simulink model "MMC_1module_twist_20251006"  (R2024b)
settings: Solver=FixedStepAuto  StartTime=t_init_sim  StopTime=sim_time  FixedStep=Ts
model workspace (MAT data in the model file):
  Phs = Simulink.Parameter
  Phs.Complexity = 'real'
  Phs.Dimensions = [0 0]
  Phs.Description = 'Phase shift of the system'
  Phs.DataType = 'auto'
  Phs.DocUnits = 'degrees'
values from neighbouring files (symbols this model uses):
  C1low1_active = 1    [script_MMC_1module_twist_20251002.m]
  C2low1_active = 1    [script_MMC_1module_twist_20251002.m]
  expdelay = 0.00798    [script_MMC_1module_twist_20251002.m]
  f_HF_test = f_HF_tab(f_index)    [script_MMC_1module_twist_20251002.m]
  feeder_current_lower_rate_limit = -10    [script_MMC_1module_twist_20251002.m]    (also in twist_parameters.m = -500)
  feeder_current_upper_rate_limit = 0.386/(20e-3)    (= 19.3)    [twist_parameters.m]
  is6VExternallySupplied = false    [script_MMC_1module_twist_20251002.m]
  isFeederJumperOpen = false    [script_MMC_1module_twist_20251002.m]
  isHighFrequencyTest = false    [script_MMC_1module_twist_20251002.m]
  power_losses = false    [script_MMC_1module_twist_20251002.m]
  power_supply_C = 62.71e-2    (= 0.6271)    [script_MMC_1module_twist_20251002.m]
  power_supply_rC_down = 7.016e-2    (= 0.07016)    [script_MMC_1module_twist_20251002.m]
  power_supply_rC_up = 0.1    [script_MMC_1module_twist_20251002.m]
  R = 15    [MMC_parameters.m]
  Rdec = 15    [MMC_parameters.m]
  source_V = 0    [script_MMC_1module_twist_20251002.m]
  Ts = 1e-6    (= 1e-06)    [script_MMC_1module_twist_20251002.m]
  twist_data_acquisition_delay = 50e-9    (= 5e-08)    [script_MMC_1module_twist_20251002.m]
  twist_data_sampling_period = 1/twist_freq_data_sampling    (= 5e-05)    [script_MMC_1module_twist_20251002.m]
  twist_dead_time = 200e-9    (= 2e-07)    [twist_parameters.m]    (also in twist_parameters_before.m)
  twist_freq_switching = 200e3    (= 200000)    [twist_parameters.m]    (also in twist_parameters_before.m)
  twist_high_side_adc_R = 1/(1/2e6 + 1/2e6 + 1/(330e3+5.6e3))    (= 251272.836178)    [twist_parameters.m]    (also in twist_parameters_before.m = 335600)
  twist_high_side_C = 33e-6*4 + 4.7e-6*12    (= 0.0001884)    [twist_parameters.m]    (also in twist_parameters_before.m)
  twist_high_side_feeder_R = 47e3+4.7e3    (= 51700)    [twist_parameters.m]
  twist_high_side_rC = 0.1    [twist_parameters.m]    (also in twist_parameters_before.m)
  twist_low_side_adc_R = 150e3+470    (= 150470)    [twist_parameters.m]    (also in twist_parameters_before.m)
  twist_low_side_C_ceramic = 3*4.7e-6    (= 1.41e-05)    [twist_parameters.m]    (also in twist_parameters_before.m)
  twist_low_side_C_electrolytic = 47e-6    (= 4.7e-05)    [twist_parameters.m]    (also in twist_parameters_before.m)
  twist_low_side_L = 33e-6    (= 3.3e-05)    [twist_parameters.m]    (also in twist_parameters_before.m)
  twist_low_side_rC = 700e-3    (= 0.7)    [twist_parameters.m]    (also in twist_parameters_before.m = 0.35)
  twist_low_side_rL = 10e-3    (= 0.01)    [twist_parameters.m]    (also in twist_parameters_before.m)
  twist_R_VCC = (tau_VCC/twist_high_side_C  - twist_high_side_rC)/(1-(tau_VCC/twist_high_side_C - twist_high_side_rC)/R_parallel)    (= 1110.74997822)    [twist_parameters.m]
  VDC = 40    [MMC_parameters.m]
  Vdc_off_time = 0.4912    [script_MMC_1module_twist_20251002.m]
  Vdc_on_time = -0.0024    [script_MMC_1module_twist_20251002.m]
undefined symbols (not defined in the file or in its folder): C_SM, feeder_current, feeder_current_tab, gcbh, L_ac, power_supply_rC, sps_rtmsupport, twist_low_side_lC
libraries: spsSeriesRLCBranchLib x17, spsVoltageMeasurementLib x8, spsCurrentMeasurementLib x6, spsTriangleGeneratorLib x6, spsMosfetLib x6, spsIdealSwitchLib x4, spsDiodeLib x3, spsControlledCurrentSourceLib x3, spsGroundLib x1, spsControlledVoltageSourceLib x1, spspowerguiLib x1
(part 1 of 2)
settings Model: Creator=rodgeur  LastModifiedBy=ana
settings SolverCC: AlgebraicLoopSolver=TrustRegion
settings DataIOCC: SaveOutput=off  DSMLogging=off
settings DebuggingCC: AlgebraicLoopMsg=none  UnconnectedInputMsg=warning  UnconnectedOutputMsg=warning  UnconnectedLineMsg=warning  ArithmeticOperatorsInVariantConditions=warning
settings ModelReferenceCC: EnableRefExpFcnMdlSchedulingChecks=on
settings SFSimCC: CustomCodeUndefinedFunction=UseInterfaceOnly
settings RTWCC: GPUComputeCapability=3.5  DLArmComputeVersion=19.05

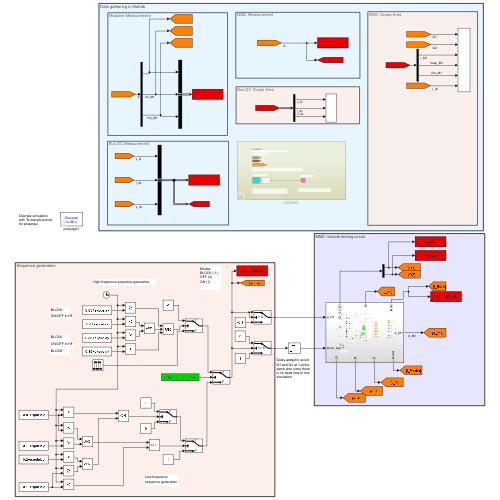
[thumbnail: Simulink's stored preview of the top-level diagram]
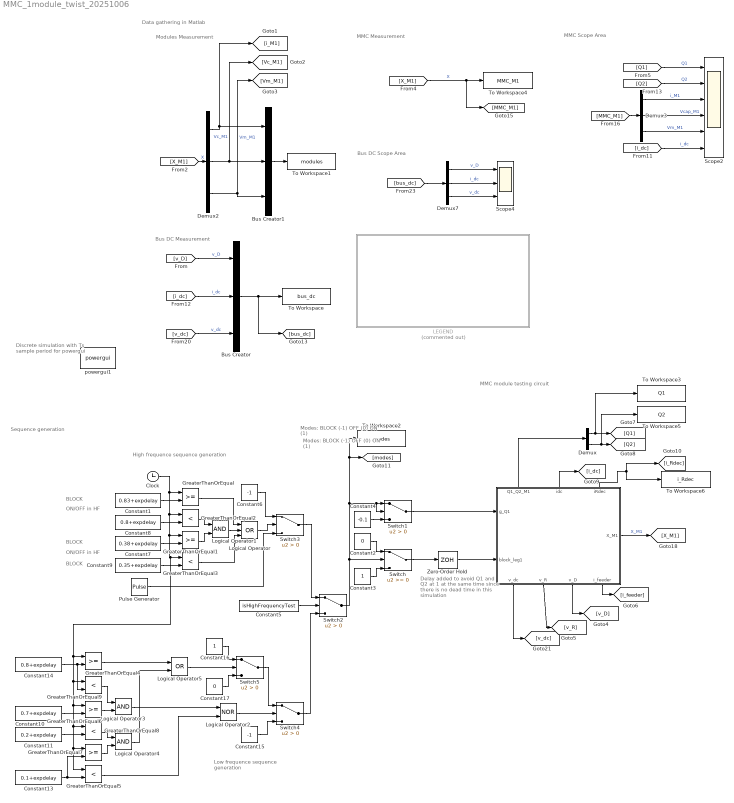
== system MMC_1module_twist_20251006 ==
  note: Modules Measurement
  note: Data gathering in Matlab
  note: MMC Measurement
  note: Bus DC Measurement
  note: MMC Scope Area
  note: MMC module testing circuit
  note: Bus DC Scope Area
  note: Sequence generation
  note: Delay added to avoid Q1 and Q2 at 1 at the same time since there is no dead time in this simulation
  note: Modes:
      | BLOCK (-1)
      | OFF (0)
      | ON (1)
  note: Modes:
      | BLOCK (-1)
      | OFF (0)
      | ON (1)
  note: High frequence sequence generation
  note: Discrete simulation with Ts sample period for powergui
  note: BLOCK
  note: BLOCK
  note: ON/OFF in HF
  note: BLOCK
  note: ON/OFF in HF
  note: Low frequence sequence generation
  " " : Subsystem
      settings: PortSchema="{\"entries\":[{\"content\":{\"sides\":[{\"content\":{\"connectorIds\":[\"In1\",\"In2\"]},\"type\":\"ConnectorPlacement.EquallySpacedRectSide\",\"uuid\":\"1684c177-0f69-459b-8ce9-190a6cc7c2f7\"},{\"content\":{\"connectorIds\":[\"Out1\"],\"side\":\"RIGHT\"},\"type\":\"ConnectorPlacement.EquallySpacedRectSide\",\"uuid\":\"0bff5431-30f2-45f3-9612-3e8ee114177b\"},{\"content\":{\"connectorIds\":[\"Out6\",\"Out7\",\"Out8\"],\"side\":\"TOP\"},\"type\":\"ConnectorPlacement.EquallySpacedRectSide\",\"uuid\":\"5880dbee-f5bf-4d11-b41f-6e883d19a036\"},{\"content\":{\"connectorIds\":[\"Out2\",\"Out3\",\"Out4\",\"Out5\"],\"side\":\"BOTTOM\"},\"type\":\"ConnectorPlacement.EquallySpacedRectSide\",\"uuid\":\"e7f28e42-6c15-4753-aad9-7fd8153dbb2b\"}]},\"type\":\"ConnectorPlacement.EquallySpacedConnector\",\"uuid\":\"d5dc9c97-4c49-4fa9-8e0e-631ade92c721\"}],\"packageUris\":[\"http://schema.mathworks.com/mf0/Connector/R2020b\"],\"version\":\"1.0\"}"
  Bus Creator : BusCreator  Inputs=3
  Bus Creator1 : BusCreator  Inputs=3
  Clock : Clock
  Constant1 : Constant  Value=0.83+expdelay
  Constant10 : Constant  Value=0.7+expdelay
  Constant11 : Constant  Value=0.2+expdelay
  Constant13 : Constant  Value=0.1+expdelay
  Constant14 : Constant  Value=0.8+expdelay
  Constant15 : Constant  Value=-1
  Constant16 : Constant
  Constant17 : Constant  Value=0
  Constant2 : Constant  Value=0
  Constant3 : Constant
  Constant4 : Constant  Value=-0.1
  Constant5 : Constant  Value=isHighFrequencyTest
  Constant6 : Constant  Value=-1
  Constant7 : Constant  Value=0.38+expdelay
  Constant8 : Constant  Value=0.8+expdelay
  Constant9 : Constant  Value=0.35+expdelay
  Demux : Demux  Outputs=2
  Demux2 : Demux  Outputs=3
  Demux3 : Demux  Outputs=3
  Demux7 : Demux  Outputs=3
  GreaterThanOrEqual{,1,4,6..7} (5 alike) : RelationalOperator  OutDataTypeStr=boolean  RndMeth=Simplest  InputSameDT=off
  GreaterThanOrEqual{2..3,5,8..9} (5 alike) : RelationalOperator  Operator=<  OutDataTypeStr=boolean  RndMeth=Simplest  InputSameDT=off
  LEGEND : Subsystem  Commented=on
  Logical Operator : Logic  Operator=OR  Inputs=3  AllPortsSameDT=off  OutDataTypeStr=boolean
  Logical Operator1 : Logic  AllPortsSameDT=off  OutDataTypeStr=boolean
  Logical Operator2 : Logic  Operator=NOR  AllPortsSameDT=off  OutDataTypeStr=boolean
  Logical Operator3 : Logic  AllPortsSameDT=off  OutDataTypeStr=boolean
  Logical Operator4 : Logic  AllPortsSameDT=off  OutDataTypeStr=boolean
  Logical Operator5 : Logic  Operator=OR  AllPortsSameDT=off  OutDataTypeStr=boolean
  Pulse Generator : DiscretePulseGenerator  Period=round(1/(f_HF_test*Ts))  PulseWidth=round(1/(f_HF_test*Ts*2))  PhaseDelay=round(((expdelay))/Ts)  SampleTime=Ts
  Scope2 : Scope  NumInputPorts=6
  Scope4 : Scope  NumInputPorts=3
  Switch : Switch  SaturateOnIntegerOverflow=off  InputSameDT=off
  Switch{1..5} (5 alike) : Switch  Criteria=u2 > Threshold  SaturateOnIntegerOverflow=off  InputSameDT=off
  To Workspace : ToWorkspace  VariableName=bus_dc  SaveFormat=Structure With Time  SampleTime=-1
  To Workspace1 : ToWorkspace  VariableName=modules  SaveFormat=Structure With Time  SampleTime=-1
  To Workspace2 : ToWorkspace  VariableName=modes  SaveFormat=Structure With Time  SampleTime=-1
  To Workspace3 : ToWorkspace  VariableName=Q1  SaveFormat=Structure With Time  SampleTime=-1
  To Workspace4 : ToWorkspace  VariableName=MMC_M1  SaveFormat=Structure With Time  SampleTime=-1
  To Workspace5 : ToWorkspace  VariableName=Q2  SaveFormat=Structure With Time  SampleTime=-1
  To Workspace6 : ToWorkspace  VariableName=i_Rdec  SaveFormat=Structure With Time  SampleTime=-1
  Zero-Order Hold : ZeroOrderHold  SampleTime=5*Ts
  powergui1 : spspowerguiLib/powergui  Priority=1  SimulationMode=Discrete  SampleTime=Ts  frequency=60  Iterations=50  frequencyindice=0  Pbase=100e6  ErrMax=1e-4  UnitsV=V  UnitsW=W  buscounter=0  FunctionMessages=off  echomessages=off  EnableUseOfTLC=off  CurrentSourceSwitches=off  DisableSnubberDevices=off  DisableRonSwitches=off  DisableVfSwitches=off  DisplayEquations=off  AutomaticDiscreteSolvers=off  SolverType=Backward Euler  Interpol=off  ExternalGateDelay=off  methode=off  Ts=0  x0status=blocks  SPID=off  SwTol=0  HookPort=off  NonlinearTolerance=1e-4  nMaxIteration=100  ContinueOnMaxIteration=off  RestoreLinks=warning  ResistiveCurrentMeasurement=off  Frange=[0:2:500]  Ylog=off  Xlog=on  ShowGrid=off  save=off  variable=ZData  structure=0  ZoomFFT=off  StartTime=0.0  cycles=1  DisplayStyle=1  fundamental=60  FreqAxis=off  MaxFrequency=1000  frequencyindicesteady=1  RmsSteady=1  display=off
  wires:
  Bus Creator1/1 -> To Workspace1/1
  Bus Creator/1 -> To Workspace/1, [bus_dc]
  [v_D] -> Bus Creator/1  "v_D"
  [v_dc] -> Bus Creator/3  "v_dc"
  [X_M1] -> [MMC_M1], To Workspace4/1  "X"
  " "/1(X_M1) -> [X_M1]  "X_M1"
  " "/2(v_dc) -> [v_dc]
  Demux3/2 -> Scope2/4  "Vcap_M1"
  Demux3/1 -> Scope2/3  "i_M1"
  Demux3/3 -> Scope2/5  "Vm_M1"
  [MMC_M1] -> Demux3/1
  [bus_dc] -> Demux7/1
  Demux7/1 -> Scope4/1  "v_D"
  Demux7/3 -> Scope4/3  "v_dc"
  [X_M1] -> Demux2/1  "X"
  Demux2/2 -> [Vc_M1], Bus Creator1/2  "Vc_M1"
  Demux2/3 -> [Vm_M1], Bus Creator1/3  "Vm_M1"
  Demux2/1 -> Bus Creator1/1, [i_M1]
  " "/3(v_R) -> [v_R]
  " "/4(v_D) -> [v_D]
  " "/5(i_feeder) -> [i_feeder]
  [i_dc] -> Scope2/6  "i_dc"
  [i_dc] -> Bus Creator/2  "i_dc"
  Demux7/2 -> Scope4/2  "i_dc"
  Constant4/1 -> Switch1/3
  Constant2/1 -> Switch/1
  Constant5/1 -> Switch2/2
  Constant3/1 -> Switch/3
  Switch2/1 -> To Workspace2/1, [modes], Switch1/2, Switch1/1, Switch/2
  Switch1/1 -> " "/1(g_Q1)
  " "/6(Q1_Q2_M1) -> Demux/1
  Demux/1 -> To Workspace3/1, [Q1]
  Demux/2 -> To Workspace5/1, [Q2]
  [Q1] -> Scope2/1  "Q1"
  [Q2] -> Scope2/2  "Q2"
  " "/7(idc) -> [i_dc]
  Pulse Generator/1 -> Switch3/3
  Constant1/1 -> GreaterThanOrEqual/2
  Constant6/1 -> Switch3/1
  Switch3/1 -> Switch2/1
  Switch4/1 -> Switch2/3
  Logical Operator/1 -> Switch3/2
  GreaterThanOrEqual/1 -> Logical Operator/1
  Logical Operator1/1 -> Logical Operator/2
  GreaterThanOrEqual1/1 -> Logical Operator1/2
  Constant7/1 -> GreaterThanOrEqual1/2
  GreaterThanOrEqual2/1 -> Logical Operator1/1
  Constant8/1 -> GreaterThanOrEqual2/2
  Switch/1 -> Zero-Order Hold/1
  Zero-Order Hold/1 -> " "/2(block_leg1)
  " "/8(iRdec) -> To Workspace6/1, [i_Rdec]
  Constant9/1 -> GreaterThanOrEqual3/2
  GreaterThanOrEqual3/1 -> Logical Operator/3
  Constant15/1 -> Switch4/3
  Switch5/1 -> Switch4/1
  Logical Operator2/1 -> Switch4/2
  Logical Operator3/1 -> Logical Operator2/1
  GreaterThanOrEqual9/1 -> Logical Operator3/1
  GreaterThanOrEqual8/1 -> Logical Operator4/1
  Constant13/1 -> GreaterThanOrEqual7/2, GreaterThanOrEqual5/2
  Constant10/1 -> GreaterThanOrEqual6/2
  Constant16/1 -> Switch5/1
  GreaterThanOrEqual7/1 -> Logical Operator4/2
  Constant11/1 -> GreaterThanOrEqual8/2
  GreaterThanOrEqual5/1 -> Logical Operator2/2
  Logical Operator4/1 -> Logical Operator5/2
  Constant14/1 -> GreaterThanOrEqual9/2, GreaterThanOrEqual4/2
  Clock/1 -> GreaterThanOrEqual2/1, GreaterThanOrEqual7/1, GreaterThanOrEqual5/1, GreaterThanOrEqual8/1, GreaterThanOrEqual6/1, GreaterThanOrEqual9/1, GreaterThanOrEqual4/1, GreaterThanOrEqual3/1, GreaterThanOrEqual1/1, GreaterThanOrEqual/1
  Constant17/1 -> Switch5/3
  GreaterThanOrEqual6/1 -> Logical Operator3/2
  Logical Operator5/1 -> Switch5/2
  GreaterThanOrEqual4/1 -> Logical Operator5/1

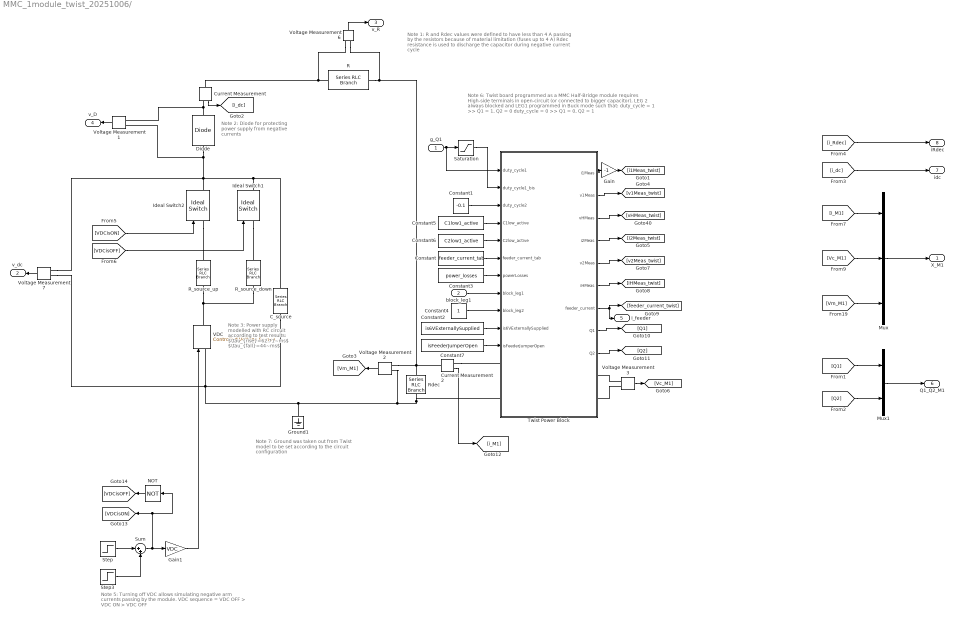
== system MMC_1module_twist_20251006/  ==
  note: Note 2:
      | Diode for protecting power supply from negative currents
  note: Note 3:
      | Power supply modelled with RC circuit according to test results:
      |
      | $\tau_{rise}=62.71~ms$
      | $\tau_{fall}=44~ms$
  note: Note 5:
      | Turning off VDC allows simulating negative arm currents passing by the module.
      |
      | VDC sequence = VDC OFF > VDC ON > VDC OFF
  note: Note 1:
      | R and Rdec values were defined to have less than 4 A passing by the resistors because of material limitation (fuses up to 4 A)
      |
      | Rdec resistance is used to discharge the capacitor during negative current cycle
  note: Note 6:
      | Twist board programmed as a MMC Half-Bridge module requires High-side terminals in open-circuit (or connected to bigger capacitor), LEG 2 always blocked and LEG1 programmed in Buck mode such that:
      |
      | duty_cycle = 1 >> Q1 = 1, Q2 = 0
      | duty_cycle = 0 >> Q1 = 0, Q2 = 1
  note: Note 7:
      | Ground was taken out from Twist model to be set according to the circuit configuration
  g_Q1 : Inport
  block_leg1 : Inport  Port=2
  C_source : spsSeriesRLCBranchLib/Series RLC Branch  LConnTagsString=__new0  RConnTagsString=__new0  BranchType=C  Resistance=power_supply_rC  Inductance=1e-3  SetiL0=off  InitialCurrent=0  Capacitance=power_supply_C  Setx0=on  InitialVoltage=0  Measurements=None
  Constant : Constant  Value=feeder_current_tab
  Constant1 : Constant  Value=-0.1
  Constant2 : Constant  Value=is6VExternallySupplied
  Constant3 : Constant  Value=power_losses
  Constant4 : Constant
  Constant5 : Constant  Value=C1low1_active
  Constant6 : Constant  Value=C2low1_active
  Constant7 : Constant  Value=isFeederJumperOpen
  Current Measurement : spsCurrentMeasurementLib/Current Measurement  PhasorSimulation=off  OutputType=Complex  PSBequivalent=0
  Current Measurement2 : spsCurrentMeasurementLib/Current Measurement  PhasorSimulation=off  OutputType=Complex  PSBequivalent=0
  Diode : spsDiodeLib/Diode  Ron=0.325  Lon=0  Vf=0.4404  IC=0  UseSnubber=0  Rs=500  Cs=250e-9  Measurements=off
  Gain : Gain  Gain=-1
  Gain1 : Gain  Gain=VDC
  Ground1 : spsGroundLib/Ground  LConnTagsString=a
  Ideal Switch1 : spsIdealSwitchLib/Ideal Switch  Ron=0.001  Lon=0  IC=0  Rs=1e5  Cs=inf  Measurements=on
  Ideal Switch2 : spsIdealSwitchLib/Ideal Switch  Ron=0.001  Lon=0  IC=0  Rs=1e5  Cs=inf  Measurements=on
  Mux : Mux  Inputs=3
  Mux1 : Mux  Inputs=2
  NOT : Logic  Operator=NOT  IconShape=distinctive  AllPortsSameDT=off  OutDataTypeStr=boolean
  R : spsSeriesRLCBranchLib/Series RLC Branch  LConnTagsString=__new0  RConnTagsString=__new0  BranchType=R  Resistance=R  Inductance=L_ac  SetiL0=off  InitialCurrent=0  Capacitance=C_SM  Setx0=off  InitialVoltage=0  Measurements=None
  R_source_down : spsSeriesRLCBranchLib/Series RLC Branch  LConnTagsString=__new0  RConnTagsString=__new0  BranchType=R  Resistance=power_supply_rC_down  Inductance=1e-3  SetiL0=off  InitialCurrent=0  Capacitance=power_supply_C  Setx0=off  InitialVoltage=0  Measurements=None
  R_source_up : spsSeriesRLCBranchLib/Series RLC Branch  LConnTagsString=__new0  RConnTagsString=__new0  BranchType=R  Resistance=power_supply_rC_up  Inductance=1e-3  SetiL0=off  InitialCurrent=0  Capacitance=power_supply_C  Setx0=off  InitialVoltage=0  Measurements=None
  Rdec : spsSeriesRLCBranchLib/Series RLC Branch  LConnTagsString=__new0  RConnTagsString=__new0  BranchType=R  Resistance=Rdec  Inductance=L_ac  SetiL0=off  InitialCurrent=0  Capacitance=C_SM  Setx0=off  InitialVoltage=0  Measurements=None
  Saturation : Saturate  UpperLimit=1  LowerLimit=0
  Step : Step  Time=Vdc_off_time  Before=1  After=0  SampleTime=0
  Step3 : Step  Time=Vdc_on_time  Before=-1  After=0  SampleTime=0
  Sum : Sum  Inputs=|++
  Twist Power Block : Subsystem
  VDC : spsControlledVoltageSourceLib/Controlled Voltage Source  Initialize=on  Source_Type=DC  Amplitude=VDC  Phase=0  Frequency=0  Measurements=None
  Voltage Measurement{1..3,6..7} (5 alike) : spsVoltageMeasurementLib/Voltage Measurement  PhasorSimulation=off  OutputType=Complex  PSBequivalent=0
  X_M1 : Outport
  v_dc : Outport  Port=2
  v_R : Outport  Port=3
  v_D : Outport  Port=4
  i_feeder : Outport  Port=5
  Q1_Q2_M1 : Outport  Port=6
  idc : Outport  Port=7
  iRdec : Outport  Port=8
  wires:
  Voltage Measurement6/1 -> v_R/1
  Voltage Measurement7/1 -> v_dc/1
  Twist Power Block/2(v1Meas) -> [v1Meas_twist]
  Constant/1 -> Twist Power Block/6(feeder_current_tab)
  Twist Power Block/7(feeder_current) -> [feeder_current_twist], i_feeder/1
  Constant3/1 -> Twist Power Block/7(powerLosses)
  Constant1/1 -> Twist Power Block/3(duty_cycle2)
  Twist Power Block/6(iHMeas) -> [iHMeas_twist]
  Twist Power Block/5(v2Meas) -> [v2Meas_twist]
  Twist Power Block/3(vHMeas) -> [vHMeas_twist]
  g_Q1/1 -> Twist Power Block/1(duty_cycle1), Saturation/1
  Saturation/1 -> Twist Power Block/2(duty_cycle1_bis)
  Twist Power Block/1(i1Meas) -> Gain/1
  Gain/1 -> [i1Meas_twist]
  Voltage Measurement1/1 -> v_D/1
  Current Measurement/1 -> [i_dc]
  Voltage Measurement2/1 -> [Vm_M1]
  Voltage Measurement3/1 -> [Vc_M1]
  [Vc_M1] -> Mux/2
  [i_M1] -> Mux/1
  [Vm_M1] -> Mux/3
  Mux/1 -> X_M1/1
  block_leg1/1 -> Twist Power Block/8(block_leg1)
  Twist Power Block/8(Q1) -> [Q1]
  Twist Power Block/9(Q2) -> [Q2]
  [Q1] -> Mux1/1
  [Q2] -> Mux1/2
  Mux1/1 -> Q1_Q2_M1/1
  Current Measurement2/1 -> [i_M1]
  [i_dc] -> idc/1
  Step/1 -> Sum/1
  Step3/1 -> Sum/2
  [i_Rdec] -> iRdec/1
  Constant2/1 -> Twist Power Block/10(is6VExternallySupplied)
  Constant4/1 -> Twist Power Block/9(block_leg2)
  Sum/1 -> NOT/1, [VDCisON], Gain1/1
  Gain1/1 -> VDC/1
  [VDCisON] -> Ideal Switch2/1
  [VDCisOFF] -> Ideal Switch1/1
  NOT/1 -> [VDCisOFF]
  Twist Power Block/4(i2Meas) -> [i2Meas_twist]
  Constant5/1 -> Twist Power Block/4(C1low_active)
  Constant6/1 -> Twist Power Block/5(C2low_active)
  Constant7/1 -> Twist Power Block/11(isFeederJumperOpen)
  connections:
  Twist Power Block/LConn3 -- Voltage Measurement2/LConn2 -- Ground1/LConn1 -- VDC/LConn1 -- Voltage Measurement7/LConn2 -- C_source/RConn1 -- Rdec/RConn1
  Voltage Measurement6/LConn1 -- Current Measurement/LConn1 -- R/LConn1
  Diode/RConn1 -- Voltage Measurement1/LConn2 -- Current Measurement/RConn1
  Voltage Measurement3/LConn1 -- Twist Power Block/RConn1
  Voltage Measurement3/LConn2 -- Twist Power Block/RConn2
  Current Measurement2/RConn1 -- Twist Power Block/LConn1
  R/RConn1 -- Voltage Measurement6/LConn2 -- Voltage Measurement2/LConn1 -- Current Measurement2/LConn1 -- Rdec/LConn1
  R_source_up/RConn1 -- R_source_down/RConn1 -- VDC/RConn1
  Diode/LConn1 -- Ideal Switch1/RConn1 -- C_source/LConn1 -- Voltage Measurement7/LConn1 -- Ideal Switch2/RConn1 -- Voltage Measurement1/LConn1
  Ideal Switch2/LConn1 -- R_source_up/LConn1
  Ideal Switch1/LConn1 -- R_source_down/LConn1

== system MMC_1module_twist_20251006/LEGEND ==
  note: Note:
      | Name the signals going into the scope to faciliate reading
  note: Color Code for scope
  note: Color code for subsystems
  note: Note:
      | Small subsystems usually contain a reduced set of functions
      | Model blocks regroup several small subsystems
  note: Note: Please avoid using global variables.  Rather, create the appropriate input/output
      | port in your subsystem
  note: This is a block for standardize the creation of models in simulink
  note: Color Code for variables
  note: LEGEND
  Model Blocks : Subsystem
  Scope : Scope
  Small subsystem : Subsystem
  wires:
  Model Blocks/1(Output_Example) -> Scope/1  "signal_name"

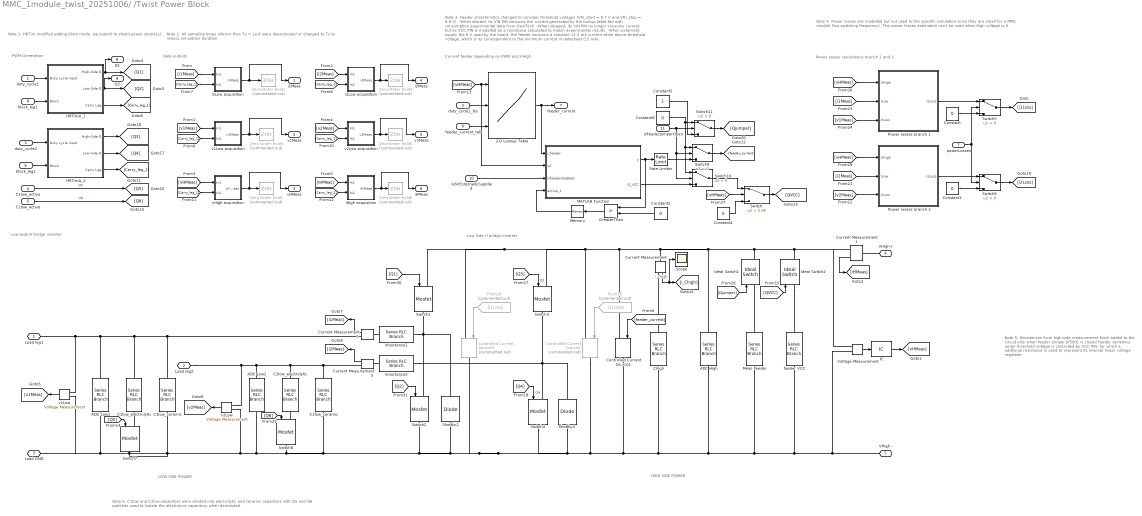
== system MMC_1module_twist_20251006/ /Twist Power Block ==
  note: Power losses calculations branch 1 and 2
  note: Current feeder depending on PWM and VHigh
  note: LOW SIDE POWER
  note: Data outputs
  note: PWM Generation
  note: Low-Side H bridge inverter
  note: Low Side H bridge inverter
  note: HIGH SIDE POWER
  note: Note 1:
      | HRTim modified adding block mode, equivalent to shield.power.stop(ALL);
  note: Note 2:
      | All sampling times inferior than Ts = 1e-6 were desactivated or changed to Ts to reduce simulation duration
  note: Note 3:
      | Feeder chracteristics changed to consider threshold voltages (Vth_start = 9.7 V and Vth_stop = 8.9 V).
      | -When started, its VIN PIN consums the current generated by the lookup table fed with consumption experimental data from OwnTech.
      | -When stopped, its VIN PIN no longer consums current but its VCC PIN is modelled as a resistance calculated to match experimental results.
      | -When externally supply the 6 V used by the board, the feeder consums a constant 11.2 mA current when above threshold voltage, which is its correspondent to the minimum current in datasheet (15 mA).
  note: Note 5:
      |
      | Resistances from high-side measurement block added to the circuit only when feeder jumper JP5001 is closed
      |
      | Feeder dynamics under threshold voltage is controlled by VCC PIN, for which a addtional resistance is used to represent its internal linear voltage regulator
  note: Note 4:
      | Power losses are modelled but not used in this specific simulation since they are small for a MMC module (low switching frequency).
      |
      | This power losses estimation can't be used when High voltage is 0.
  note: Note 6:
      | C1low and C2low capacitors were divided into electrolytic and ceramic capacitors with Q5 and Q6 switches used to isolate the electrolytic capacitors when demanded.
  duty_cycle1 : Inport
  duty_cycle1_bis : Inport  Port=2
  duty_cycle2 : Inport  Port=3
  C1low_active : Inport  Port=4
  C2low_active : Inport  Port=5
  feeder_current_tab : Inport  Port=6
  powerLosses : Inport  Port=7
  block_leg1 : Inport  Port=8
  block_leg2 : Inport  Port=9
  is6VExternallySupplied : Inport  Port=10
  isFeederJumperOpen : Inport  Port=11
  2-D Lookup Table : Lookup_n-D  LookupTableObject=feeder_current_tab  BreakpointsSpecification=Even spacing  BreakpointsForDimension1=[1:4]  BreakpointsForDimension2=[1:3]  BreakpointsForDimension1FirstPoint=feeder_VHigh_min  BreakpointsForDimension2FirstPoint=feeder_duty_min  BreakpointsForDimension1Spacing=feeder_VHigh_spacing  BreakpointsForDimension2Spacing=feeder_duty_spacing  TableSource=Input port  Table=feeder_current  InternalRulePriority=Speed  RndMeth=Simplest
      settings: InputPortMap=u0,u1,p221
  ADC High : spsSeriesRLCBranchLib/Series RLC Branch  LConnTagsString=__new0  RConnTagsString=__new0  BranchType=R  Resistance=twist_high_side_adc_R  Inductance=twist_low_side_L  SetiL0=off  InitialCurrent=0  Capacitance=1e-6  Setx0=off  InitialVoltage=0  Measurements=None
  ADC Low1 : spsSeriesRLCBranchLib/Series RLC Branch  LConnTagsString=__new0  RConnTagsString=__new0  BranchType=R  Resistance=twist_low_side_adc_R  Inductance=twist_low_side_L  SetiL0=off  InitialCurrent=0  Capacitance=1e-6  Setx0=off  InitialVoltage=0  Measurements=Branch voltage
  ADC Low2 : spsSeriesRLCBranchLib/Series RLC Branch  LConnTagsString=__new0  RConnTagsString=__new0  BranchType=R  Resistance=twist_low_side_adc_R  Inductance=twist_low_side_L  SetiL0=off  InitialCurrent=0  Capacitance=1e-6  Setx0=off  InitialVoltage=0  Measurements=Branch voltage
  C1low_ceramic : spsSeriesRLCBranchLib/Series RLC Branch  LConnTagsString=__new0  RConnTagsString=__new0  BranchType=C  Resistance=twist_low_side_rC  Inductance=1e-3  SetiL0=off  InitialCurrent=0  Capacitance=twist_low_side_C_ceramic  Setx0=off  InitialVoltage=0  Measurements=None
  C1low_electrolytic : spsSeriesRLCBranchLib/Series RLC Branch  LConnTagsString=__new0  RConnTagsString=__new0  BranchType=RC  Resistance=twist_low_side_rC  Inductance=twist_low_side_lC  SetiL0=off  InitialCurrent=0  Capacitance=twist_low_side_C_electrolytic  Setx0=off  InitialVoltage=0  Measurements=None
  C2low_ceramic : spsSeriesRLCBranchLib/Series RLC Branch  LConnTagsString=__new0  RConnTagsString=__new0  BranchType=C  Resistance=twist_low_side_rC  Inductance=1e-3  SetiL0=off  InitialCurrent=0  Capacitance=twist_low_side_C_ceramic  Setx0=off  InitialVoltage=0  Measurements=None
  C2low_electrolytic : spsSeriesRLCBranchLib/Series RLC Branch  LConnTagsString=__new0  RConnTagsString=__new0  BranchType=RC  Resistance=twist_low_side_rC  Inductance=twist_low_side_lC  SetiL0=off  InitialCurrent=0  Capacitance=twist_low_side_C_electrolytic  Setx0=off  InitialVoltage=0  Measurements=None
  Chigh : spsSeriesRLCBranchLib/Series RLC Branch  LConnTagsString=__new0  RConnTagsString=__new0  BranchType=RC  Resistance=twist_high_side_rC  Inductance=1e-3  SetiL0=off  InitialCurrent=0  Capacitance=twist_high_side_C  Setx0=on  InitialVoltage=source_V  Measurements=None
  Constant{,1..2,4,6} (5 alike) : Constant  Value=0
  Constant5 : Constant
  Controlled Current Source1 : spsControlledCurrentSourceLib/Controlled Current Source  Initialize=on  Source_Type=AC  Amplitude=0  Phase=0  Frequency=0  Measurements=None
  Controlled Current Source2 : spsControlledCurrentSourceLib/Controlled Current Source  Commented=on  Initialize=on  Source_Type=AC  Amplitude=0  Phase=0  Frequency=0  Measurements=None
  Controlled Current Source3 : spsControlledCurrentSourceLib/Controlled Current Source  Commented=on  Initialize=on  Source_Type=AC  Amplitude=0  Phase=0  Frequency=0  Measurements=None
  Current Measurement{,1,5..6} (4 alike) : spsCurrentMeasurementLib/Current Measurement  PhasorSimulation=off  OutputType=Complex  PSBequivalent=0
  From16 : From  Commented=on  GotoTag=i2Loss
  From28 : From  Commented=on  GotoTag=i1Loss
  GreaterThan : RelationalOperator  Operator=>  OutDataTypeStr=boolean  RndMeth=Simplest  InputSameDT=off
  HRTimA_1 : Subsystem
  HRTimA_2 : Subsystem
  IC : InitialCondition  Value=source_V
  Ideal Switch1 : spsIdealSwitchLib/Ideal Switch  Ron=0.001  Lon=0  IC=0  Rs=1e5  Cs=inf  Measurements=on
  Ideal Switch2 : spsIdealSwitchLib/Ideal Switch  Ron=0.001  Lon=0  IC=0  Rs=1e5  Cs=inf  Measurements=on
  Inductance1 : spsSeriesRLCBranchLib/Series RLC Branch  LConnTagsString=__new0  RConnTagsString=__new0  BranchType=RL  Resistance=twist_low_side_rL  Inductance=twist_low_side_L  SetiL0=off  InitialCurrent=0  Capacitance=1e-6  Setx0=off  InitialVoltage=0  Measurements=None
  Inductance2 : spsSeriesRLCBranchLib/Series RLC Branch  LConnTagsString=__new0  RConnTagsString=__new0  BranchType=RL  Resistance=twist_low_side_rL  Inductance=twist_low_side_L  SetiL0=off  InitialCurrent=0  Capacitance=1e-6  Setx0=off  InitialVoltage=0  Measurements=None
  MATLAB Function : MATLAB Function  TreatAsAtomicUnit=on
  Meas Feeder : spsSeriesRLCBranchLib/Series RLC Branch  LConnTagsString=__new0  RConnTagsString=__new0  BranchType=R  Resistance=twist_high_side_feeder_R  Inductance=twist_low_side_L  SetiL0=off  InitialCurrent=0  Capacitance=1e-6  Setx0=off  InitialVoltage=0  Measurements=None
  Memory : Memory  InheritSampleTime=on  LinearizeAsDelay=on
  Power losses branch 1 : Subsystem
  Power losses branch 2 : Subsystem
  Rate Limiter : RateLimiter  RisingSlewLimit=feeder_current_upper_rate_limit  FallingSlewLimit=feeder_current_lower_rate_limit  SampleTimeMode=inherited
  Scope : Scope
  Shottky2 : spsDiodeLib/Diode  Ron=twist_shottky_Ron  Lon=0  Vf=twist_shottky_Vf  IC=0  UseSnubber=0  Rs=twist_shottky_Rs  Cs=twist_shottky_Cs  Measurements=off
  Shottky4 : spsDiodeLib/Diode  Ron=twist_shottky_Ron  Lon=0  Vf=twist_shottky_Vf  IC=0  UseSnubber=0  Rs=twist_shottky_Rs  Cs=twist_shottky_Cs  Measurements=off
  Switch : Switch  Criteria=u2 > Threshold  Threshold=2.05  SaturateOnIntegerOverflow=off  InputSameDT=off
  Switch{1..4} (4 alike) : spsMosfetLib/Mosfet  Ron=twist_FET_Ron  Lon=0  Rd=twist_FET_Rd  Vfd=twist_FET_Vf  IC=0  Rs=twist_FET_Rs  Cs=twist_FET_Cs  Measurements=off
  Switch{5..6,9..11} (5 alike) : Switch  Criteria=u2 > Threshold  SaturateOnIntegerOverflow=off  InputSameDT=off
  Switch7 : spsMosfetLib/Mosfet  Ron=twist_FET_Clow_Ron  Lon=0  Rd=twist_FET_Clow_Ron  Vfd=0  IC=0  Rs=twist_FET_Rs  Cs=twist_FET_Cs  Measurements=off
  Switch8 : spsMosfetLib/Mosfet  Ron=twist_FET_Clow_Ron  Lon=0  Rd=twist_FET_Clow_Ron  Vfd=0  IC=0  Rs=twist_FET_Rs  Cs=twist_FET_Cs  Measurements=off
  Voltage Measurement : spsVoltageMeasurementLib/Voltage Measurement  PhasorSimulation=off  OutputType=Complex  PSBequivalent=0
  Zero-Order Hold{1..6} (6 alike) : ZeroOrderHold  Commented=on  SampleTime=twist_data_sampling_period
  feeder VCC : spsSeriesRLCBranchLib/Series RLC Branch  LConnTagsString=__new0  RConnTagsString=__new0  BranchType=R  Resistance=twist_R_VCC  Inductance=twist_low_side_L  SetiL0=off  InitialCurrent=0  Capacitance=1e-6  Setx0=off  InitialVoltage=0  Measurements=None
  i1Low acquisition : Subsystem
  i2Low acquisition : Subsystem
  iHigh acquisition : Subsystem
  v1Low : spsVoltageMeasurementLib/Voltage Measurement  PhasorSimulation=off  OutputType=Complex  PSBequivalent=0
  v1Low acquisition : Subsystem
  v2Low : spsVoltageMeasurementLib/Voltage Measurement  PhasorSimulation=off  OutputType=Complex  PSBequivalent=0
  v2Low acquisition : Subsystem
  vHigh acquisition : Subsystem
  Load leg1 : PMIOPort  Side=Left
  Load leg2 : PMIOPort  Port=2  Side=Left
  Load GND : PMIOPort  Port=3  Side=Left
  VHigh+ : PMIOPort  Port=4  Side=Right
  VHigh - : PMIOPort  Port=5  Side=Right
  i1Meas : Outport
  v1Meas : Outport  Port=2
  vHMeas : Outport  Port=3
  i2Meas : Outport  Port=4
  v2Meas : Outport  Port=5
  iHMeas : Outport  Port=6
  feeder_current : Outport  Port=7
  Q1 : Outport  Port=8
  Q2 : Outport  Port=9
  wires:
  duty_cycle1/1 -> HRTimA_1/1(Duty cycle input)
  HRTimA_1/2(Low-Side Q) -> [Q2], Q2/1
  [v1Meas] -> v1Low acquisition/1(In1)
  C1low_active/1 -> [Q5]  "Q5"
  HRTimA_1/1(High-Side Q) -> [Q1], Q1/1
  HRTimA_2/1(High-Side Q) -> [Q3]
  HRTimA_2/2(Low-Side Q) -> [Q4]
  [Carry_leg_1] -> vHigh acquisition/2(In2)
  [vHMeas] -> vHigh acquisition/1(In1)
  [i2Meas] -> i2Low acquisition/1(In1)
  [Carry_leg_2] -> i2Low acquisition/2(In2)
  [v2Meas] -> v2Low acquisition/1(In1)
  [Carry_leg_2] -> v2Low acquisition/2(In2)
  [iHMeas] -> iHigh acquisition/1(In1)
  [Carry_leg_2] -> iHigh acquisition/2(In2)
  [Carry_leg_1] -> v1Low acquisition/2(In2)
  v1Low acquisition/1(v1Meas) -> v1Meas/1, Zero-Order Hold3/1
  i2Low acquisition/1(i2Meas) -> i2Meas/1, Zero-Order Hold4/1
  v2Low acquisition/1(v2Meas) -> v2Meas/1, Zero-Order Hold5/1
  iHigh acquisition/1(iHMeas) -> iHMeas/1, Zero-Order Hold6/1
  vHigh acquisition/1(vHMeas) -> vHMeas/1, Zero-Order Hold2/1
  HRTimA_2/3(Carry Leg) -> [Carry_leg_2]
  HRTimA_1/3(Carry Leg) -> [Carry_leg_1]
  duty_cycle2/1 -> HRTimA_2/1(Duty cycle input)
  [vHMeas] -> MATLAB Function/2(vC), 2-D Lookup Table/1
  v2Low/1 -> [v2Meas]
  [Q3] -> Switch3/1  "Q3"
  Current Measurement6/1 -> [i1Meas]
  [Q1] -> Switch1/1
  [Q4] -> Switch4/1  "Q4"
  v1Low/1 -> [v1Meas]
  [Q2] -> Switch2/1
  Current Measurement1/1 -> [iHMeas]
  Current Measurement5/1 -> [i2Meas]
  [Carry_leg_1] -> i1Low acquisition/2(In2)
  [i1Meas] -> i1Low acquisition/1(In1)
  i1Low acquisition/1(i1Meas) -> i1Meas/1, Zero-Order Hold1/1
  Voltage Measurement/1 -> IC/1
  IC/1 -> [vHMeas]
  [vHMeas] -> Power losses branch 1/1(VHigh)
  [i1Meas] -> Power losses branch 1/2(ILow)
  [v1Meas] -> Power losses branch 1/3(VLow)
  Power losses branch 1/1(i1Loss) -> Switch5/1
  Switch5/1 -> [i1Loss]
  Constant/1 -> Switch5/3
  feeder_current_tab/1 -> 2-D Lookup Table/3
  duty_cycle1_bis/1 -> 2-D Lookup Table/2
  [Q5] -> Switch7/1
  C2low_active/1 -> [Q6]  "Q6"
  [feeder_current] -> Controlled Current Source1/1
  block_leg1/1 -> HRTimA_1/2(Block)
  Current Measurement/1 -> Scope/1, [i_Chigh]  "i_Chigh"
  block_leg2/1 -> HRTimA_2/2(Block)
  GreaterThan/1 -> Memory/1
  Constant2/1 -> GreaterThan/2
  [QVCC] -> Ideal Switch2/1
  2-D Lookup Table/1 -> feeder_current/1, MATLAB Function/1(i_feeder)
  MATLAB Function/1(y) -> GreaterThan/1, Rate Limiter/1
  powerLosses/1 -> Switch5/2, Switch6/2
  [vHMeas] -> Power losses branch 2/1(VHigh)
  [i2Meas] -> Power losses branch 2/2(ILow)
  [v2Meas] -> Power losses branch 2/3(VLow)
  Switch6/1 -> [i2Loss]
  Constant1/1 -> Switch6/3
  Power losses branch 2/1(i1Loss) -> Switch6/1
  is6VExternallySupplied/1 -> MATLAB Function/3(isfeederdisabled)
  Memory/1 -> MATLAB Function/4(active_1)
  [vHMeas] -> Switch/2
  Constant4/1 -> Switch/3
  [Q6] -> Switch8/1
  Switch9/1 -> [feeder_current]
  Rate Limiter/1 -> Switch9/3
  MATLAB Function/2(Q_VCC) -> Switch10/3
  Constant6/1 -> Switch11/1, Switch10/1, Switch9/1
  isFeederJumperOpen/1 -> Switch11/2, Switch9/2, Switch10/2
  Switch/1 -> [QVCC]
  Switch10/1 -> Switch/1
  Constant5/1 -> Switch11/3
  Switch11/1 -> [Qjumper]
  [Qjumper] -> Ideal Switch1/1
  From16/1 -> Controlled Current Source2/1
  From28/1 -> Controlled Current Source3/1
  connections:
  Inductance2/LConn1 -- Current Measurement5/LConn1
  Current Measurement6/LConn1 -- Inductance1/LConn1
  VHigh+/RConn1 -- Current Measurement1/LConn1
  v2Low/LConn1 -- Load leg2/RConn1 -- ADC Low2/LConn1 -- C2low_electrolytic/LConn1 -- C2low_ceramic/LConn1 -- Current Measurement5/RConn1
  Switch4/LConn1 -- Switch3/RConn1 -- Shottky4/RConn1 -- Inductance2/RConn1
  v1Low/LConn1 -- Load leg1/RConn1 -- C1low_ceramic/LConn1 -- Current Measurement6/RConn1 -- C1low_electrolytic/LConn1 -- ADC Low1/LConn1
  Current Measurement/RConn1 -- Chigh/LConn1
  ADC High/RConn1 -- Meas Feeder/RConn1 -- feeder VCC/RConn1 -- Voltage Measurement/LConn2 -- VHigh -/RConn1 -- Chigh/RConn1 -- Controlled Current Source2/RConn1 -- Controlled Current Source3/RConn1 -- Switch2/RConn1 -- Load GND/RConn1 -- v1Low/LConn2 -- ADC Low1/RConn1 -- Switch7/RConn1 -- C1low_ceramic/RConn1 -- v2Low/LConn2 -- ADC Low2/RConn1 -- Switch8/RConn1 -- C2low_ceramic/RConn1 -- Shottky2/LConn1 -- Switch4/RConn1 -- Shottky4/LConn1 -- Controlled Current Source1/RConn1
  Switch7/LConn1 -- C1low_electrolytic/RConn1
  Switch8/LConn1 -- C2low_electrolytic/RConn1
  Inductance1/RConn1 -- Shottky2/RConn1 -- Switch2/LConn1 -- Switch1/RConn1
  Ideal Switch2/LConn1 -- feeder VCC/LConn1
  Current Measurement/LConn1 -- Ideal Switch1/RConn1 -- Voltage Measurement/LConn1 -- Current Measurement1/RConn1 -- Ideal Switch2/RConn1 -- ADC High/LConn1 -- Controlled Current Source2/LConn1 -- Controlled Current Source3/LConn1 -- Switch1/LConn1 -- Switch3/LConn1 -- Controlled Current Source1/LConn1
  Meas Feeder/LConn1 -- Ideal Switch1/LConn1

== system MMC_1module_twist_20251006/LEGEND/Model Blocks ==
  Output_Example : Outport

== system MMC_1module_twist_20251006/LEGEND/Small subsystem ==

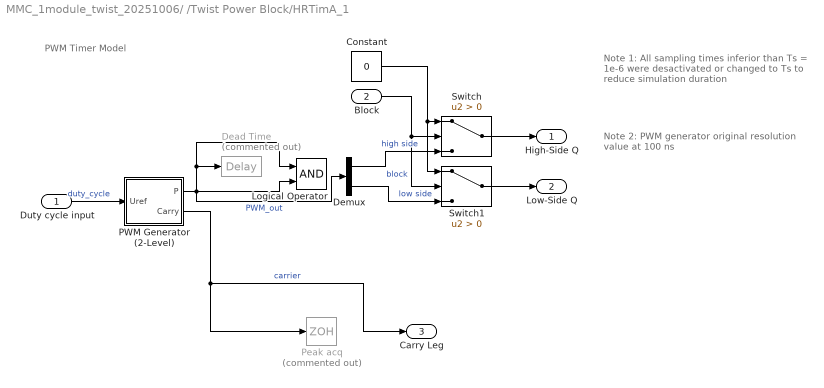
== system MMC_1module_twist_20251006/ /Twist Power Block/HRTimA_1 ==
  note: PWM Timer Model
  note: Note 1:
      | All sampling times inferior than Ts = 1e-6 were desactivated or changed to Ts to reduce simulation duration
  note: Note 2:
      | PWM generator original resolution value at 100 ns
  Duty cycle input : Inport
  Block : Inport  Port=2
  Constant : Constant  Value=0
  Dead Time : TransportDelay  Commented=on  DelayTime=twist_dead_time
  Demux : Demux  Outputs=2
  Logical Operator : Logic  AllPortsSameDT=off  OutDataTypeStr=boolean
  PWM Generator (2-Level) : Subsystem  AncestorBlock=|  DialogController=POWERSYS.PowerSysDialog  LoadFcn=sps_rtmsupport('LoadFcn', gcbh);  StartFcn=sps_rtmsupport('StartFcn', gcbh);  StopFcn=sps_rtmsupport('StopFcn', gcbh);  BlockChoice=InternalUref  mask(PWM Generator (2-Level)){ModulatorType=Single-phase half-bridge (2 pulses), ModulatorMode=Unsynchronized, Fc=twist_freq_switching, Pc=0, nF=27, MinMax=[0 1], SamplingTechnique=Symmetrical regular (single edge), ModulatingSignals=off, m=0.8, Freq=60, Phase=0, Ts=Ts, ShowCarrierOutport=off}
      | spsPWMGenerator2LevelLib/PWM Generator
      | (2-Level)
      mask prompts: ModulatorType "Generator type:"; ModulatorMode "Mode of operation:"; Fc "Frequency (Hz):"; Pc "Initial phase (degrees):"; nF "Switching ratio (carrier frequency / output frequency):"; MinMax "Minimum and maximum values: [ Min  Max ]"; SamplingTechnique "Sampling technique:"; ModulatingSignals "Internal generation of reference signal"; m "Modulation index:"; Freq "Frequency (Hz):"; Phase "Phase (degrees):"; Ts "Sample time (s):"; ShowCarrierOutport "Show measurement port"
      mask help:
      | Generate pulses for PWM-controlled 2-Level converter, using carrier-based two-level PWM method. The block can control switching devices of single-phase half-bridge, single-phase full-bridge (unipolar or bipolar modulation) or three-phase bridge.
      |
      | When the Synchronized mode of operation is selected, a second input is added to the block, and the internal generation of modulating signal is disabled. Use input 2 (wt) to synchronize the carrier.
      mask init:
      | sps = powericon('PWMGenerator2LevelInit',gcb,ModulatorType,SamplingTechnique,ModulatorMode,nF,Fc,MinMax,Pc,ShowCarrierOutport,ModulatingSignals,m,Freq,Phase,Ts);
      settings: CopyFcn=sps_rtmsupport('CopyFcn', gcbh);  DeleteFcn=sps_rtmsupport('DeleteFcn', gcbh);  UndoDeleteFcn=sps_rtmsupport('UndoDeleteFcn', gcbh);  ModelCloseFcn=sps_rtmsupport('ModelCloseFcn', gcbh);  PreSaveFcn=sps_rtmsupport('PreSaveFcn', gcbh);  PostSaveFcn=sps_rtmsupport('PostSaveFcn', gcbh);  NameChangeFcn=sps_rtmsupport('NameChangeFcn', gcbh);  PreCopyFcn=sps_rtmsupport('PreCopyFcn', gcbh);  OpenFcn="sps_rtmsupport('OpenFcn', gcbh, [1   2   7   8  13]);"  CloseFcn=sps_rtmsupport('CloseFcn', gcbh);  PreDeleteFcn=sps_rtmsupport('PreDeleteFcn', gcbh);
      mask Help: helpview(psbhelp);
      mask TypeOptions ModulatorType: Single-phase half-bridge (2 pulses) | Single-phase full-bridge (4 pulses) | Single-phase full-bridge - Bipolar modulation (4 pulses) | Three-phase bridge (6 pulses)
      mask TypeOptions ModulatorMode: Synchronized | Unsynchronized
      mask Callback ModulatorMode: powericon('PWMGenerator2LevelCback',gcb);
      mask TypeOptions SamplingTechnique: Natural | Asymmetrical regular (double edge) | Symmetrical regular (single edge)
      mask Callback ModulatingSignals: powericon('PWMGenerator2LevelCback',gcb);
      mask DialogControl Container3 Prompt: Carrier
      mask DialogControl ModulatingSignalParameters Prompt: Reference signal
  Peak acq : ZeroOrderHold  Commented=on  SampleTime=twist_data_acquisition_delay
  Switch : Switch  Criteria=u2 > Threshold  SaturateOnIntegerOverflow=off  InputSameDT=off
  Switch1 : Switch  Criteria=u2 > Threshold  SaturateOnIntegerOverflow=off  InputSameDT=off
  High-Side Q : Outport
  Low-Side Q : Outport  Port=2
  Carry Leg : Outport  Port=3
  wires:
  Demux/1 -> Switch/3  "high side"
  Duty cycle input/1 -> PWM Generator (2-Level)/1(Uref)  "duty_cycle"
  PWM Generator (2-Level)/2(Carry) -> Carry Leg/1, Peak acq/1  "carrier"
  Block/1 -> Switch/2, Switch1/2  "block"
  Demux/2 -> Switch1/3  "low side"
  Switch1/1 -> Low-Side Q/1
  Switch/1 -> High-Side Q/1
  Constant/1 -> Switch1/1, Switch/1
  PWM Generator (2-Level)/1(P) -> Demux/1, Dead Time/1, Logical Operator/1, Logical Operator/2  "PWM_out"

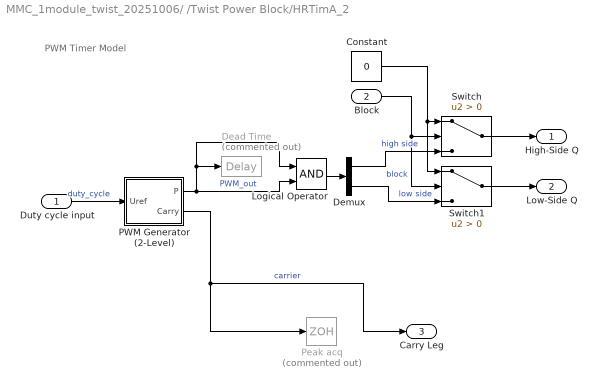
== system MMC_1module_twist_20251006/ /Twist Power Block/HRTimA_2 ==
  note: PWM Timer Model
  Duty cycle input : Inport
  Block : Inport  Port=2
  Constant : Constant  Value=0
  Dead Time : TransportDelay  Commented=on  DelayTime=twist_dead_time
  Demux : Demux  Outputs=2
  Logical Operator : Logic  AllPortsSameDT=off  OutDataTypeStr=boolean
  PWM Generator (2-Level) : Subsystem  AncestorBlock=|  DialogController=POWERSYS.PowerSysDialog  LoadFcn=sps_rtmsupport('LoadFcn', gcbh);  StartFcn=sps_rtmsupport('StartFcn', gcbh);  StopFcn=sps_rtmsupport('StopFcn', gcbh);  BlockChoice=InternalUref  mask(PWM Generator (2-Level)){ModulatorType=Single-phase half-bridge (2 pulses), ModulatorMode=Unsynchronized, Fc=twist_freq_switching, Pc=0, nF=27, MinMax=[0 1], SamplingTechnique=Symmetrical regular (single edge), ModulatingSignals=off, m=0.8, Freq=60, Phase=0, Ts=Ts, ShowCarrierOutport=off}
      | spsPWMGenerator2LevelLib/PWM Generator
      | (2-Level)
      mask prompts: ModulatorType "Generator type:"; ModulatorMode "Mode of operation:"; Fc "Frequency (Hz):"; Pc "Initial phase (degrees):"; nF "Switching ratio (carrier frequency / output frequency):"; MinMax "Minimum and maximum values: [ Min  Max ]"; SamplingTechnique "Sampling technique:"; ModulatingSignals "Internal generation of reference signal"; m "Modulation index:"; Freq "Frequency (Hz):"; Phase "Phase (degrees):"; Ts "Sample time (s):"; ShowCarrierOutport "Show measurement port"
      mask help:
      | Generate pulses for PWM-controlled 2-Level converter, using carrier-based two-level PWM method. The block can control switching devices of single-phase half-bridge, single-phase full-bridge (unipolar or bipolar modulation) or three-phase bridge.
      |
      | When the Synchronized mode of operation is selected, a second input is added to the block, and the internal generation of modulating signal is disabled. Use input 2 (wt) to synchronize the carrier.
      mask init:
      | sps = powericon('PWMGenerator2LevelInit',gcb,ModulatorType,SamplingTechnique,ModulatorMode,nF,Fc,MinMax,Pc,ShowCarrierOutport,ModulatingSignals,m,Freq,Phase,Ts);
      settings: CopyFcn=sps_rtmsupport('CopyFcn', gcbh);  DeleteFcn=sps_rtmsupport('DeleteFcn', gcbh);  UndoDeleteFcn=sps_rtmsupport('UndoDeleteFcn', gcbh);  ModelCloseFcn=sps_rtmsupport('ModelCloseFcn', gcbh);  PreSaveFcn=sps_rtmsupport('PreSaveFcn', gcbh);  PostSaveFcn=sps_rtmsupport('PostSaveFcn', gcbh);  NameChangeFcn=sps_rtmsupport('NameChangeFcn', gcbh);  PreCopyFcn=sps_rtmsupport('PreCopyFcn', gcbh);  OpenFcn="sps_rtmsupport('OpenFcn', gcbh, [1   2   7   8  13]);"  CloseFcn=sps_rtmsupport('CloseFcn', gcbh);  PreDeleteFcn=sps_rtmsupport('PreDeleteFcn', gcbh);
      mask Help: helpview(psbhelp);
      mask TypeOptions ModulatorType: Single-phase half-bridge (2 pulses) | Single-phase full-bridge (4 pulses) | Single-phase full-bridge - Bipolar modulation (4 pulses) | Three-phase bridge (6 pulses)
      mask TypeOptions ModulatorMode: Synchronized | Unsynchronized
      mask Callback ModulatorMode: powericon('PWMGenerator2LevelCback',gcb);
      mask TypeOptions SamplingTechnique: Natural | Asymmetrical regular (double edge) | Symmetrical regular (single edge)
      mask Callback ModulatingSignals: powericon('PWMGenerator2LevelCback',gcb);
      mask DialogControl Container3 Prompt: Carrier
      mask DialogControl ModulatingSignalParameters Prompt: Reference signal
  Peak acq : ZeroOrderHold  Commented=on  SampleTime=twist_data_acquisition_delay
  Switch : Switch  Criteria=u2 > Threshold  SaturateOnIntegerOverflow=off  InputSameDT=off
  Switch1 : Switch  Criteria=u2 > Threshold  SaturateOnIntegerOverflow=off  InputSameDT=off
  High-Side Q : Outport
  Low-Side Q : Outport  Port=2
  Carry Leg : Outport  Port=3
  wires:
  Logical Operator/1 -> Demux/1
  Demux/1 -> Switch/3  "high side"
  Duty cycle input/1 -> PWM Generator (2-Level)/1(Uref)  "duty_cycle"
  PWM Generator (2-Level)/2(Carry) -> Carry Leg/1, Peak acq/1  "carrier"
  Block/1 -> Switch/2, Switch1/2  "block"
  Demux/2 -> Switch1/3  "low side"
  Switch1/1 -> Low-Side Q/1
  Switch/1 -> High-Side Q/1
  Constant/1 -> Switch1/1, Switch/1
  PWM Generator (2-Level)/1(P) -> Dead Time/1, Logical Operator/1, Logical Operator/2  "PWM_out"

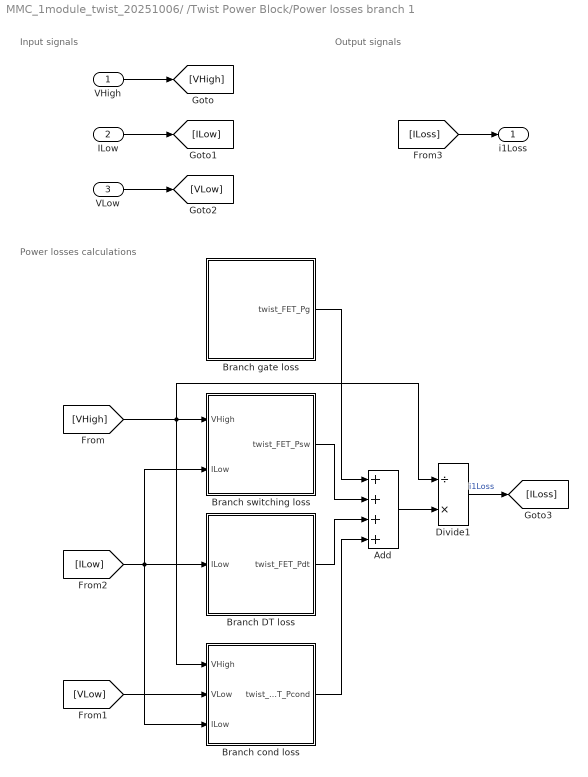
== system MMC_1module_twist_20251006/ /Twist Power Block/Power losses branch 1 ==
  note: Output signals
  note: Input signals
  note: Power losses calculations
  VHigh : Inport
  ILow : Inport  Port=2
  VLow : Inport  Port=3
  Add : Sum  Inputs=++++
  Branch DT loss : MATLAB Function  TreatAsAtomicUnit=on
  Branch cond loss : MATLAB Function  TreatAsAtomicUnit=on
  Branch gate loss : MATLAB Function  TreatAsAtomicUnit=on
  Branch switching loss : MATLAB Function  TreatAsAtomicUnit=on
  Divide1 : Product  Inputs=/*
  i1Loss : Outport
  wires:
  Branch switching loss/1(twist_FET_Psw) -> Add/2
  [ILow] -> Branch switching loss/2(ILow), Branch cond loss/3(ILow), Branch DT loss/1(ILow)
  Branch gate loss/1(twist_FET_Pg) -> Add/1
  Branch cond loss/1(twist_FET_Pcond) -> Add/4
  [VHigh] -> Divide1/1, Branch cond loss/1(VHigh), Branch switching loss/1(VHigh)
  Branch DT loss/1(twist_FET_Pdt) -> Add/3
  [VLow] -> Branch cond loss/2(VLow)
  Divide1/1 -> [ILoss]  "i1Loss"
  VHigh/1 -> [VHigh]
  ILow/1 -> [ILow]
  VLow/1 -> [VLow]
  [ILoss] -> i1Loss/1
  Add/1 -> Divide1/2

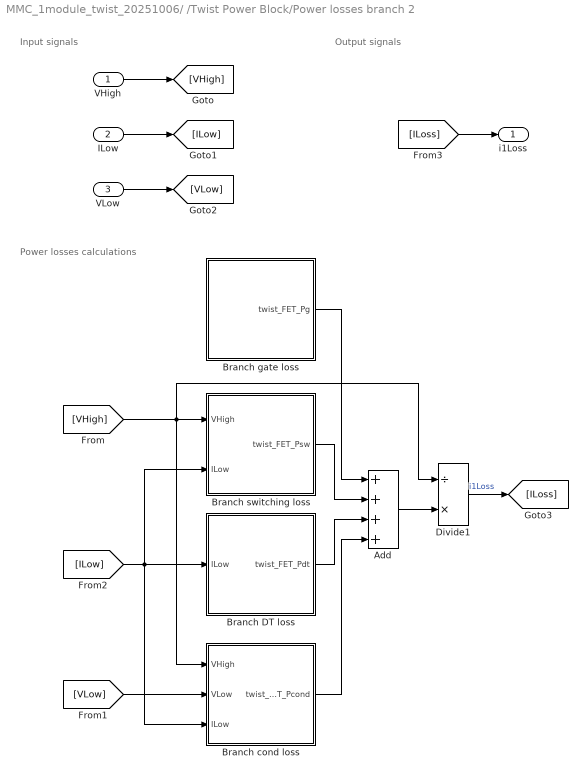
== system MMC_1module_twist_20251006/ /Twist Power Block/Power losses branch 2 ==
  note: Output signals
  note: Input signals
  note: Power losses calculations
  VHigh : Inport
  ILow : Inport  Port=2
  VLow : Inport  Port=3
  Add : Sum  Inputs=++++
  Branch DT loss : MATLAB Function  TreatAsAtomicUnit=on
  Branch cond loss : MATLAB Function  TreatAsAtomicUnit=on
  Branch gate loss : MATLAB Function  TreatAsAtomicUnit=on
  Branch switching loss : MATLAB Function  TreatAsAtomicUnit=on
  Divide1 : Product  Inputs=/*
  i1Loss : Outport
  wires:
  Branch switching loss/1(twist_FET_Psw) -> Add/2
  [ILow] -> Branch switching loss/2(ILow), Branch cond loss/3(ILow), Branch DT loss/1(ILow)
  Branch gate loss/1(twist_FET_Pg) -> Add/1
  Branch cond loss/1(twist_FET_Pcond) -> Add/4
  [VHigh] -> Divide1/1, Branch cond loss/1(VHigh), Branch switching loss/1(VHigh)
  Branch DT loss/1(twist_FET_Pdt) -> Add/3
  [VLow] -> Branch cond loss/2(VLow)
  Divide1/1 -> [ILoss]  "i1Loss"
  VHigh/1 -> [VHigh]
  ILow/1 -> [ILow]
  VLow/1 -> [VLow]
  [ILoss] -> i1Loss/1
  Add/1 -> Divide1/2

== system MMC_1module_twist_20251006/ /Twist Power Block/i1Low acquisition ==
  In1 : Inport
  In2 : Inport  Port=2
  If : If  IfExpression=u1 > 0.99  ShowElse=off
  If Action Subsystem : Subsystem  TreatAsAtomicUnit=on
  Scope : Scope  NumInputPorts=3
  i1Meas : Outport
  wires:
  If Action Subsystem/1(Out1) -> Scope/1, i1Meas/1  "Data_Carry"
  In1/1 -> Scope/2, If Action Subsystem/1(In1)  "Data"
  If/1 -> If Action Subsystem/Action
  In2/1 -> If/1, Scope/3  "Carry"

== system MMC_1module_twist_20251006/ /Twist Power Block/i2Low acquisition ==
  In1 : Inport
  In2 : Inport  Port=2
  If : If  IfExpression=u1 > 0.99  ShowElse=off
  If Action Subsystem : Subsystem  TreatAsAtomicUnit=on
  Scope : Scope  NumInputPorts=3
  i2Meas : Outport
  wires:
  If Action Subsystem/1(Out1) -> Scope/1, i2Meas/1  "Data_Carry"
  In1/1 -> Scope/2, If Action Subsystem/1(In1)  "Data"
  If/1 -> If Action Subsystem/Action
  In2/1 -> If/1, Scope/3  "Carry"

== system MMC_1module_twist_20251006/ /Twist Power Block/iHigh acquisition ==
  In1 : Inport
  In2 : Inport  Port=2
  If : If  IfExpression=u1 > 0.99  ShowElse=off
  If Action Subsystem : Subsystem  TreatAsAtomicUnit=on
  Scope : Scope  NumInputPorts=3
  iHMeas : Outport
  wires:
  If Action Subsystem/1(Out1) -> Scope/1, iHMeas/1  "Data_Carry"
  In1/1 -> Scope/2, If Action Subsystem/1(In1)  "Data"
  If/1 -> If Action Subsystem/Action
  In2/1 -> If/1, Scope/3  "Carry"

== system MMC_1module_twist_20251006/ /Twist Power Block/v1Low acquisition ==
  In1 : Inport
  In2 : Inport  Port=2
  If : If  IfExpression=u1 > 0.99  ShowElse=off
  If Action Subsystem : Subsystem  TreatAsAtomicUnit=on
  Scope : Scope  NumInputPorts=3
  v1Meas : Outport
  wires:
  If Action Subsystem/1(Out1) -> Scope/1, v1Meas/1  "Data_Carry"
  In1/1 -> Scope/2, If Action Subsystem/1(In1)  "Data"
  If/1 -> If Action Subsystem/Action
  In2/1 -> If/1, Scope/3  "Carry"

== system MMC_1module_twist_20251006/ /Twist Power Block/v2Low acquisition ==
  In1 : Inport
  In2 : Inport  Port=2
  If : If  IfExpression=u1 > 0.99  ShowElse=off
  If Action Subsystem : Subsystem  TreatAsAtomicUnit=on
  Scope : Scope  NumInputPorts=3
  v2Meas : Outport
  wires:
  If Action Subsystem/1(Out1) -> Scope/1, v2Meas/1  "Data_Carry"
  In1/1 -> Scope/2, If Action Subsystem/1(In1)  "Data"
  If/1 -> If Action Subsystem/Action
  In2/1 -> If/1, Scope/3  "Carry"

== system MMC_1module_twist_20251006/ /Twist Power Block/vHigh acquisition ==
  In1 : Inport
  In2 : Inport  Port=2
  If : If  IfExpression=u1 > 0.99  ShowElse=off
  If Action Subsystem : Subsystem  TreatAsAtomicUnit=on
  Scope : Scope  NumInputPorts=3
  vHMeas : Outport
  wires:
  If Action Subsystem/1(Out1) -> Scope/1, vHMeas/1  "Data_Carry"
  In1/1 -> Scope/2, If Action Subsystem/1(In1)  "Data"
  If/1 -> If Action Subsystem/Action
  In2/1 -> If/1, Scope/3  "Carry"
